simulink model "model"  (R2026a)
settings: Solver=VariableStepAuto
undefined symbols (not defined in the file or in its folder): K

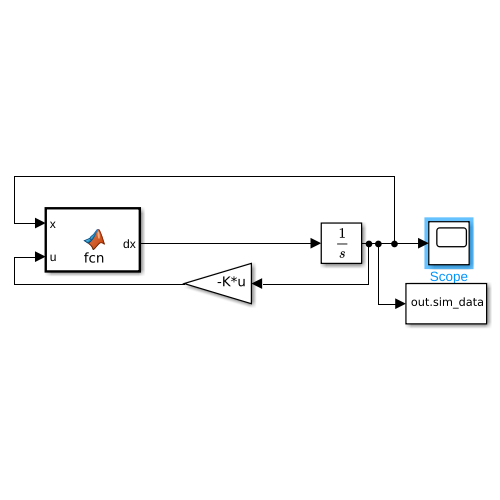
[thumbnail: Simulink's stored preview of the top-level diagram]
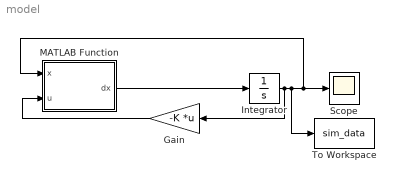
== system model ==
  Gain : Gain  Gain=-K  Multiplication=Matrix(K*u)
  Integrator : Integrator  InitialCondition=[0; 0; 0.45; 0]
  MATLAB Function : MATLAB Function  TreatAsAtomicUnit=on
  Scope : Scope
      settings: ActiveDisplayYMinimum=-21.970969882882954  ActiveDisplayYMaximum=22.901678954935026
  To Workspace : ToWorkspace  VariableName=sim_data  SampleTime=-1
  wires:
  Integrator/1 -> Scope/1, MATLAB Function/1(x), To Workspace/1, Gain/1
  Gain/1 -> MATLAB Function/2(u)
  MATLAB Function/1(dx) -> Integrator/1

== matlab function model/MATLAB Function ==
  data: x input; u input; dx output
function dx = fcn(x, u)
% 1. Force Simulink to recognize dimensions (Breaks the feedback loop confusion)
assert(all(size(x) == [4 1])); % Tells Simulink x is a 4-element column vector
assert(all(size(u) == [1 1])); % Tells Simulink u is a single scalar torque

% 2. Physical parameters
M = 1.5; m = 0.2; R = 0.05; l = 0.15; Ib = 0.012; g = 9.81; b = 0.05;

% 3. Extract states
theta = x(3); 
thetadot = x(4);

Sx = sin(theta); 
Cx = cos(theta);

% 4. Non-linear equations
denom = Ib + M*l^2 * (1 - Cx^2);

xddot = (u/R - b*x(2) + M*l*g*Sx*Cx - M*l*thetadot^2*Sx) / (M + m);
thetaddot = (M*g*l*Sx - M*l*xddot*Cx) / denom;

% 5. Output derivative vector
dx = [x(2); xddot; x(4); thetaddot];
end
